simulink model "robot_tracker"  (R2025b)
settings: Solver=VariableStepAuto  StartTime=0.0  StopTime=3.98  RelTol=1e-3
values from neighbouring files (symbols this model uses):
  Kd = 2    [main_gui_final.m]    (also in main_gui_final2.m)
  Kp = 10    [main_gui_final.m]    (also in main_gui_final2.m)
undefined symbols (not defined in the file or in its folder): L1_sim, L2_sim
settings Model: Creator=himan  LastModifiedBy=himan
settings RTWCC: GPUComputeCapability=3.5

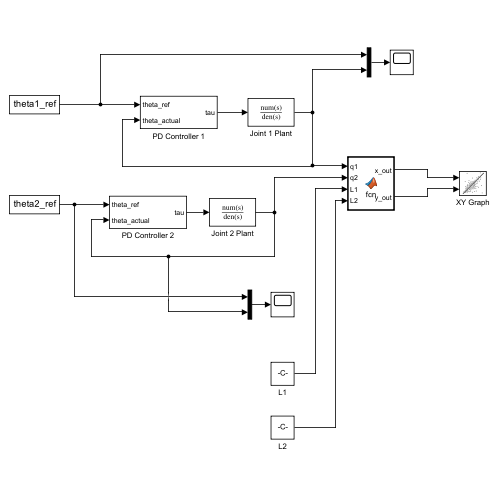
[thumbnail: Simulink's stored preview of the top-level diagram]
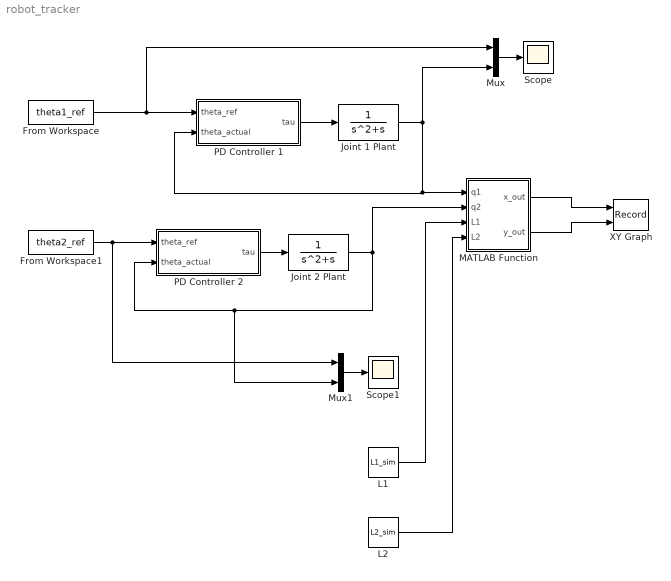
== system robot_tracker ==
  From Workspace : FromWorkspace  VariableName=theta1_ref
  From Workspace1 : FromWorkspace  VariableName=theta2_ref
  Joint 1 Plant : TransferFcn  Denominator=[1 1 0]
  Joint 2 Plant : TransferFcn  Denominator=[1 1 0]
  L1 : Constant  Value=L1_sim  SampleTime=-1
  L2 : Constant  Value=L2_sim  SampleTime=-1
  MATLAB Function : MATLAB Function  TreatAsAtomicUnit=on
  Mux : Mux  Inputs=2
  Mux1 : Mux  Inputs=2
  PD Controller 1 : Subsystem
  PD Controller 2 : Subsystem
  Scope : Scope
      settings: ActiveDisplayYMinimum=-0.95016267235405028  ActiveDisplayYMaximum=8.5514640511864553
  Scope1 : Scope
      settings: ActiveDisplayYMinimum=-3.482710840713013  ActiveDisplayYMaximum=0.38696787119033466
  XY Graph : Record  NumPorts=2.0  FileSettingsInternal="{\"entries\":[{\"content\":{\"excelSettings\":{\"content\":{},\"type\":\"Streamout.ExcelSettings\"},\"parquetSettings\":{\"content\":{},\"type\":\"Streamout.ParquetSettings\"}},\"type\":\"Streamout.FileSettingStorage\",\"uuid\":\"\"}],\"packageUris\":[\"http:\\/\\/schema.mathworks.com\\/mf0\\/streamout_blocks\\/R2020a\"],\"version\":\"1.0\"}"  FrameSettings=[0, 0]  Layout=[1 1]  SignalsInternal="{\"entries\":[{\"content\":{\"signals\":[{\"content\":{\"blockPath\":[],\"dimensions\":[1,3],\"domain\":\"\",\"hasChildren\":true,\"lineColor\":\"#edb120\",\"lineWidth\":2,\"port\":1,\"signalID\":1,\"signalName\":\"MATLAB Function:1\"},\"type\":\"RecordBlkView.Signal\",\"uuid\":\"\"},{\"content\":{\"blockPath\":[],\"channel\":[1,1],\"dimensions\":[1,3],\"domain\":\"\",\"lineColor\":\"#b746ff\",\"lineWidth\":2,\"parentID\":1,\"plots\":[ 1 ],\"port\":1,\"signalID\":2,\"signalName\":\"MATLAB Function:1\"},\"type\":\"RecordBlkView.Signal\",\"uuid\":\"\"},{\"content\":{\"blockPath\":[],\"channel\":[1,2],\"dimensions\":[1,3],\"domain\":\"\",\"lineColor\":\"#fe330a\",\"lineWidth\":2,\"parentID\":1,\"plots\":[ 1 ],\"port\":1,\"signalID\":3,\"signalName\":\"MATLAB Function:1\"},\"type\":\"RecordBlkView.Signal\",\"uuid\":\"\"},{\"content\":{\"blockPath\":[],\"channel\":[1,3],\"dimensions\":[1,3],\"domain\":\"\",\"lineColor\":\"#22b573\",\"lineWidth\":2,\"parentID\":1,\"plots\":[ 1 ],\"port\":1,\"signalID\":4,\"signalName\":\"MATLAB Function:1\"},\"type\":\"RecordBlkView.Signal\",\"uuid\":\"\"},{\"content\":{\"blockPath\":[],\"dimensions\":[1,3],\"domain\":\"\",\"hasChildren\":true,\"lineColor\":\"#77ac30\",\"lineWidth\":2,\"port\":2,\"signalID\":5,\"signalName\":\"MATLAB Function:2\"},\"type\":\"RecordBlkView.Signal\",\"uuid\":\"\"},{\"content\":{\"blockPath\":[],\"channel\":[1,1],\"dimensions\":[1,3],\"domain\":\"\",\"lineColor\":\"#ff13a6\",\"lineWidth\":2,\"parentID\":5,\"plots\":[ 1 ],\"port\":2,\"signalID\":6,\"signalName\":\"MATLAB Function:2\"},\"type\":\"RecordBlkView.Signal\",\"uuid\":\"\"},{\"content\":{\"blockPath\":[],\"channel\":[1,2],\"dimensions\":[1,3],\"domain\":\"\",\"lineColor\":\"#0072bd\",\"lineWidth\":2,\"parentID\":5,\"plots\":[ 1 ],\"port\":2,\"signalID\":7,\"signalName\":\"MATLAB Function:2\"},\"type\":\"RecordBlkView.Signal\",\"uuid\":\"\"},{\"content\":{\"blockPath\":[],\"channel\":[1,3],\"dimensions\":[1,3],\"domain\":\"\",\"lineColor\":\"#d95319\",\"lineWidth\":2,\"parentID\":5,\"plots\":[ 1 ],\"port\":2,\"signalID\":8,\"signalName\":\"MATLAB Function:2\"},\"type\":\"RecordBlkView.Signal\",\"uuid\":\"\"}]},\"type\":\"RecordBlkView.InputSignals\",\"uuid\":\"\"}],\"packageUris\":[\"http:\\/\\/schema.mathworks.com\\/mf0\\/streamout_blocks\\/R2020a\"],\"version\":\"1.0\"}"  VisualizationBindings="{\"xyplotplugin\":{\"info\":[{\"series\":[{\"bindingParametersList\":[{\"parameter\":\"X-Axis\",\"signalID\":2,\"signalName\":\"MATLAB Function:1(1,1)\"},{\"parameter\":\"Y-Axis\",\"signalID\":6,\"signalName\":\"MATLAB Function:2(1,1)\"}],\"seriesID\":0},{\"bindingParametersList\":[{\"parameter\":\"X-Axis\",\"signalID\":3,\"signalName\":\"MATLAB Function:1(1,2)\"},{\"parameter\":\"Y-Axis\",\"signalID\":7,\"signalName\":\"MATLAB Function:2(1,2)\"}],\"seriesID\":1},{\"bindingParametersList\":[{\"parameter\":\"X-Axis\",\"signalID\":4,\"signalName\":\"MATLAB Function:1(1,3)\"},{\"parameter\":\"Y-Axis\",\"signalID\":8,\"signalName\":\"MATLAB Function:2(1,3)\"}],\"seriesID\":2}],\"subplotID\":1}]}}"  CompatibilityTag=XY
  wires:
  From Workspace/1 -> Mux/1, PD Controller 1/1(theta_ref)
  PD Controller 1/1(tau) -> Joint 1 Plant/1
  Joint 1 Plant/1 -> MATLAB Function/1(q1), PD Controller 1/2(theta_actual), Mux/2
  From Workspace1/1 -> Mux1/1, PD Controller 2/1(theta_ref)
  PD Controller 2/1(tau) -> Joint 2 Plant/1
  Joint 2 Plant/1 -> Mux1/2, PD Controller 2/2(theta_actual), MATLAB Function/2(q2)
  L1/1 -> MATLAB Function/3(L1)
  L2/1 -> MATLAB Function/4(L2)
  Mux1/1 -> Scope1/1
  Mux/1 -> Scope/1
  MATLAB Function/1(x_out) -> XY Graph/1
  MATLAB Function/2(y_out) -> XY Graph/2

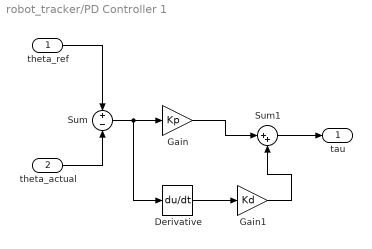
== system robot_tracker/PD Controller 1 ==
  theta_ref : Inport
  theta_actual : Inport  Port=2
  Derivative : Derivative
  Gain : Gain  Gain=Kp
  Gain1 : Gain  Gain=Kd
  Sum : Sum  Inputs=+-
  Sum1 : Sum  Inputs=|++
  tau : Outport
  wires:
  theta_ref/1 -> Sum/1
  theta_actual/1 -> Sum/2
  Sum/1 -> Derivative/1, Gain/1
  Derivative/1 -> Gain1/1
  Gain/1 -> Sum1/1
  Gain1/1 -> Sum1/2
  Sum1/1 -> tau/1

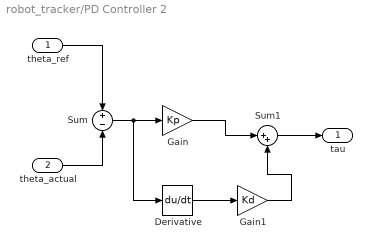
== system robot_tracker/PD Controller 2 ==
  theta_ref : Inport
  theta_actual : Inport  Port=2
  Derivative : Derivative
  Gain : Gain  Gain=Kp
  Gain1 : Gain  Gain=Kd
  Sum : Sum  Inputs=+-
  Sum1 : Sum  Inputs=|++
  tau : Outport
  wires:
  theta_ref/1 -> Sum/1
  theta_actual/1 -> Sum/2
  Sum/1 -> Derivative/1, Gain/1
  Derivative/1 -> Gain1/1
  Gain/1 -> Sum1/1
  Gain1/1 -> Sum1/2
  Sum1/1 -> tau/1

== matlab function robot_tracker/MATLAB Function ==
  data: q1 input; x_out output; q2 input; y_out output; L1 input; L2 input
% Change the first line to this:
function [x_out, y_out] = fcn(q1, q2, L1, L2)

    % REMOVE the old lines:
    % L1 = 1.0;
    % L2 = 1.0;

    % The rest of the code is the same
    x0 = 0; y0 = 0;
    x1 = L1*cos(q1);
    y1 = L1*sin(q1);
    x2 = x1 + L2*cos(q1+q2);
    y2 = y1 + L2*sin(q1+q2);
    x_out = [x0, x1, x2];
    y_out = [y0, y1, y2];
end
